simulink model "My_Nonlinear"  (R2021b)
settings: Solver=VariableStepAuto  StartTime=0.0  StopTime=simTime  RelTol=1e-3
undefined symbols (not defined in the file): b, D, g, k, L, m, MoI, p, p_dot, RPM, TakeStep, Theta
settings Model: Creator=tanzc  LastModifiedBy=tanzc

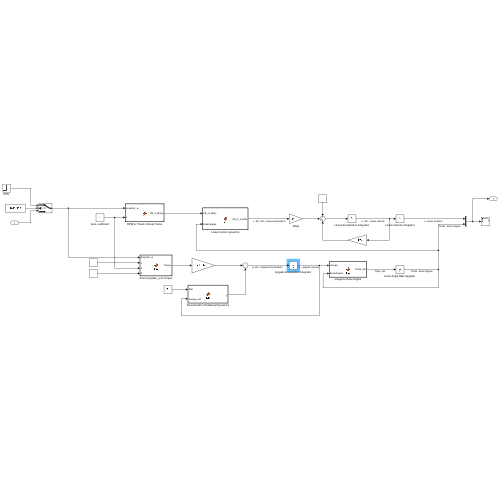
[thumbnail: Simulink's stored preview of the top-level diagram]
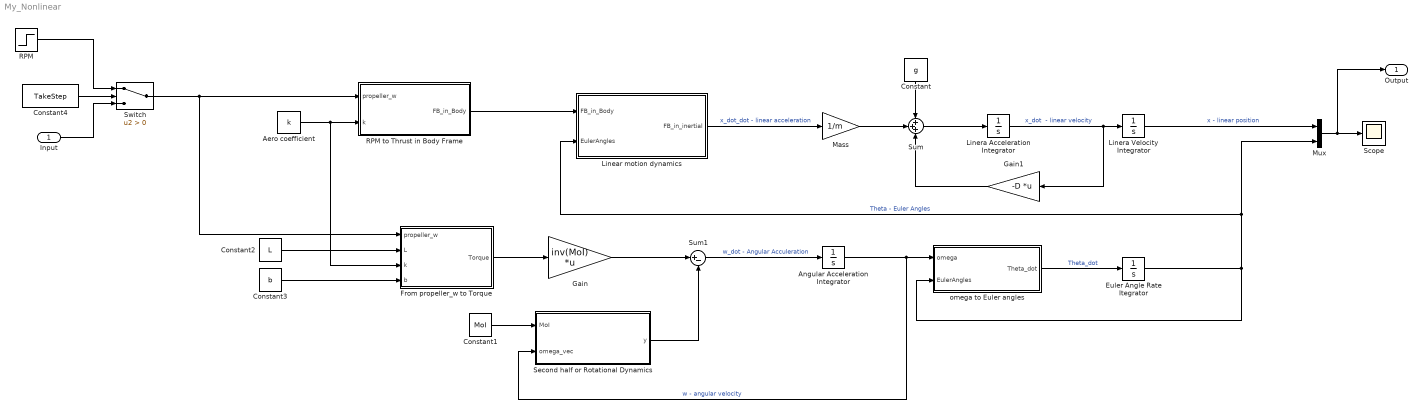
== system My_Nonlinear ==
  Input : Inport
  Aero coefficient : Constant  Value=k
  Angular Acceleration Integrator : Integrator  Priority=4  ContinuousStateAttributes='Angular_acceleration'
  Constant : Constant  Value=g
  Constant1 : Constant  Value=MoI
  Constant2 : Constant  Value=L
  Constant3 : Constant  Value=b
  Constant4 : Constant  Value=TakeStep
  Euler Angle Rate Itegrator : Integrator  Priority=3  InitialCondition=Theta  ContinuousStateAttributes='Euler_Angles'
  From propeller_w to Torque : MATLAB Function  TreatAsAtomicUnit=on
  Gain : Gain  Gain=inv(MoI)  Multiplication=Matrix(K*u)
  Gain1 : Gain  Gain=-D  Multiplication=Matrix(K*u)
  Linear motion dynamics : MATLAB Function  TreatAsAtomicUnit=on
  Linera Acceleration Integrator : Integrator  Priority=2  InitialCondition=p_dot  ContinuousStateAttributes='linear_velocity'
  Linera Velocity Integrator : Integrator  Priority=1  InitialCondition=p  ContinuousStateAttributes='linear_position'
  Mass : Gain  Gain=1/m
  Mux : Mux  Inputs=2
  RPM : Step  After=RPM  SampleTime=0
  RPM to Thrust in Body Frame : MATLAB Function  TreatAsAtomicUnit=on
  Scope : Scope
  Second half or Rotational Dynamics : MATLAB Function  TreatAsAtomicUnit=on
  Sum : Sum  Inputs=+++
  Sum1 : Sum  Inputs=|+-
  Switch : Switch  Criteria=u2 > Threshold
  omega to Euler angles : MATLAB Function  TreatAsAtomicUnit=on
  Output : Outport
  wires:
  Linear motion dynamics/1(FB_in_inertial) -> Mass/1  "x_dot_dot - linear acceleration"
  Linera Acceleration Integrator/1 -> Gain1/1, Linera Velocity Integrator/1  "x_dot  - linear velocity"
  Linera Velocity Integrator/1 -> Mux/1  "x - linear position"
  Mass/1 -> Sum/2
  Sum/1 -> Linera Acceleration Integrator/1
  Constant/1 -> Sum/1
  Gain1/1 -> Sum/3
  RPM to Thrust in Body Frame/1(FB_in_Body) -> Linear motion dynamics/1(FB_in_Body)
  Aero coefficient/1 -> From propeller_w to Torque/3(k), RPM to Thrust in Body Frame/2(k)
  From propeller_w to Torque/1(Torque) -> Gain/1
  Second half or Rotational Dynamics/1(y) -> Sum1/2
  Gain/1 -> Sum1/1
  Sum1/1 -> Angular Acceleration Integrator/1  "w_dot - Angular Acculeration"
  Angular Acceleration Integrator/1 -> Second half or Rotational Dynamics/2(omega_vec), omega to Euler angles/1(omega)  "w - angular velocity"
  omega to Euler angles/1(Theta_dot) -> Euler Angle Rate Itegrator/1  "Theta_dot"
  Euler Angle Rate Itegrator/1 -> Mux/2, Linear motion dynamics/2(EulerAngles), omega to Euler angles/2(EulerAngles)  "Theta - Euler Angles"
  Mux/1 -> Output/1, Scope/1
  Constant1/1 -> Second half or Rotational Dynamics/1(MoI)
  Constant2/1 -> From propeller_w to Torque/2(L)
  Constant3/1 -> From propeller_w to Torque/4(b)
  Switch/1 -> From propeller_w to Torque/1(propeller_w), RPM to Thrust in Body Frame/1(propeller_w)
  Constant4/1 -> Switch/2
  RPM/1 -> Switch/1
  Input/1 -> Switch/3

== matlab function My_Nonlinear/RPM to Thrust in Body Frame ==
  data: propeller_w input; FB_in_Body output; k input
function FB_in_Body = fcn(propeller_w, k)
FB_in_Body = k * [0; 0; propeller_w'*propeller_w];

== matlab function My_Nonlinear/Linear motion dynamics ==
  data: FB_in_Body input; FB_in_inertial output; EulerAngles input
function FB_in_inertial = fcn(FB_in_Body, EulerAngles)

phi = EulerAngles(1);
theta = EulerAngles(2);
psi = EulerAngles(3);

rotmZYX = eul2rotm([psi, theta, phi]);


FB_in_inertial = rotmZYX * FB_in_Body;

== matlab function My_Nonlinear/Second half or Rotational Dynamics ==
  data: MoI input; y output; omega_vec input
function y = fcn(MoI, omega_vec)
Ixx = MoI(1,1);
Iyy = MoI(2,2);
Izz = MoI(3,3);

omega_x = omega_vec(1);
omega_y = omega_vec(2);
omega_z = omega_vec(3);


y = [(Iyy - Izz)/Ixx * omega_y * omega_z;...
     (Izz-Ixx)/Iyy*omega_x*omega_z; ...
     (Ixx-Iyy)/Izz*omega_x*omega_y];

== matlab function My_Nonlinear/From propeller_w to Torque ==
  data: propeller_w input; Torque output; L input; k input; b input
function Torque = fcn(propeller_w, L, k, b)

% output:
% Torque [3x1] Vector

w1 =propeller_w(1);
w2 =propeller_w(2);
w3 =propeller_w(3);
w4 =propeller_w(4);

Torque = [ L * k * (w1^2 - w3^2);
           L * k * (w2^2 - w4^2);
           b * (w1^2 - w2^2 + w3^2 - w4^2)];

== matlab function My_Nonlinear/omega to Euler angles ==
  data: omega input; Theta_dot output; EulerAngles input
function Theta_dot = fcn(omega, EulerAngles)

phi = EulerAngles(1);
theta = EulerAngles(2);
psi = EulerAngles(3);

B = [ 1, 0, -sin(theta); ...
      0, cos(phi), cos(theta)*sin(phi); ...
      0, -sin(phi), cos(theta)*cos(phi)];
  
Theta_dot = pinv(B)*omega;
